simulink model "AsteroidImpact"  (R2021b)
settings: Solver=ode4  StartTime=0.0  StopTime=45  FixedStep=0.2  RelTol=1e-3
settings Model: Creator=KNMALE002  LastModifiedBy=lbaat
settings SolverCC: AlgebraicLoopSolver=TrustRegion
settings DataIOCC: SaveOutput=off  SignalLogging=off  DSMLogging=off  ReturnWorkspaceOutputs=off  TimeSaveName=simulation_time
settings DebuggingCC: SFMachineParentedDataDiag=warning  ArithmeticOperatorsInVariantConditions=warning
settings SFSimCC: CustomCodeUndefinedFunction=UseInterfaceOnly

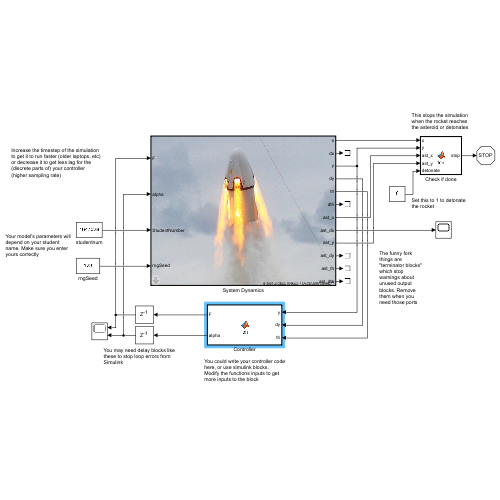
[thumbnail: Simulink's stored preview of the top-level diagram]
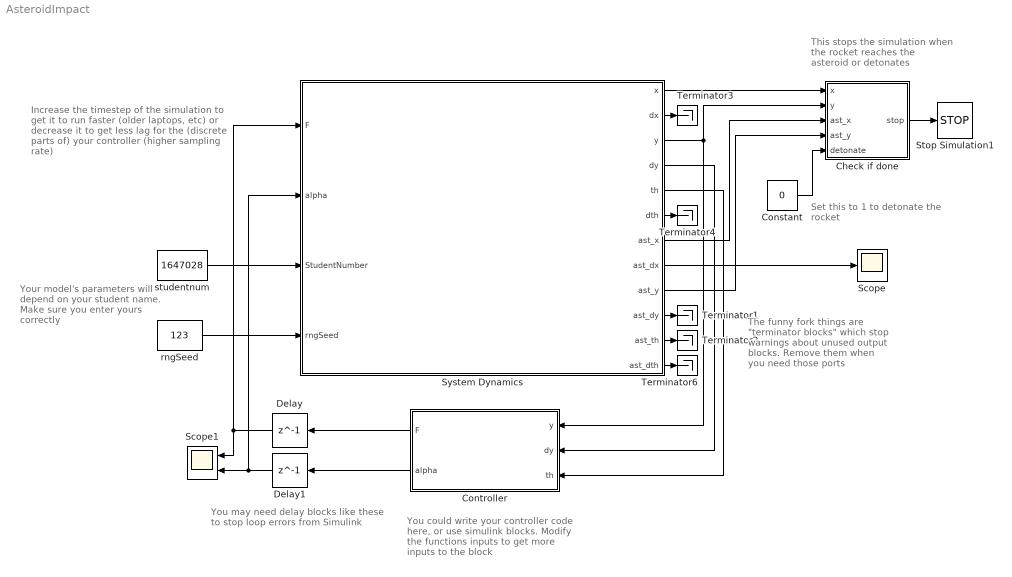
== system AsteroidImpact ==
  note: Increase the timestep of the simulation to get it to run faster (older laptops, etc) or decrease it to get less lag for the (discrete parts of) your controller (higher sampling rate)
  note: You may need delay blocks like these to stop loop errors from Simulink
  note: Your model's parameters will depend on your student name. Make sure you enter yours correctly
  note: You could write your controller code here, or use simulink blocks. Modify the functions inputs to get more inputs to the block
  note: The funny fork things are "terminator blocks" which stop warnings about unused output blocks. Remove them when you need those ports
  note: This stops the simulation when the rocket reaches the asteroid or detonates
  note: Set this to 1 to detonate the rocket
  Check if done : MATLAB Function  TreatAsAtomicUnit=on
  Constant : Constant  Value=0
  Controller : MATLAB Function  TreatAsAtomicUnit=on
  Delay : Delay  DelayLength=1  InitialCondition=10000000000
  Delay1 : Delay  DelayLength=1
  Scope : Scope
  Scope1 : Scope  NumInputPorts=2
  Stop Simulation1 : Stop
  System Dynamics : Subsystem  TreatAsAtomicUnit=on  mask{Value=1}
      mask prompts: Value "Enter mode (1, 2 or 3)"
      mask TypeOptions Value: ScenarioVar/Value
      mask Display: image('lander.jpg');
  Terminator{1..4,6} (5 alike) : Terminator
  rngSeed : Constant  Value=123
  studentnum : Constant  Value=1647028
  wires:
  studentnum/1 -> System Dynamics/3(StudentNumber)
  System Dynamics/1(x) -> Check if done/1(x)
  rngSeed/1 -> System Dynamics/4(rngSeed)
  System Dynamics/3(y) -> Check if done/2(y), Controller/1(y)
  System Dynamics/12(ast_dth) -> Terminator6/1
  System Dynamics/7(ast_x) -> Check if done/3(ast_x)
  System Dynamics/9(ast_y) -> Check if done/4(ast_y)
  System Dynamics/8(ast_dx) -> Scope/1
  System Dynamics/11(ast_th) -> Terminator2/1
  Check if done/1(stop) -> Stop Simulation1/1
  Delay1/1 -> Scope1/2, System Dynamics/2(alpha)
  Delay/1 -> Scope1/1, System Dynamics/1(F)
  Controller/1(F) -> Delay/1
  Controller/2(alpha) -> Delay1/1
  Constant/1 -> Check if done/5(detonate)
  System Dynamics/4(dy) -> Controller/2(dy)
  System Dynamics/5(th) -> Controller/3(th)
  System Dynamics/10(ast_dy) -> Terminator1/1
  System Dynamics/2(dx) -> Terminator3/1
  System Dynamics/6(dth) -> Terminator4/1

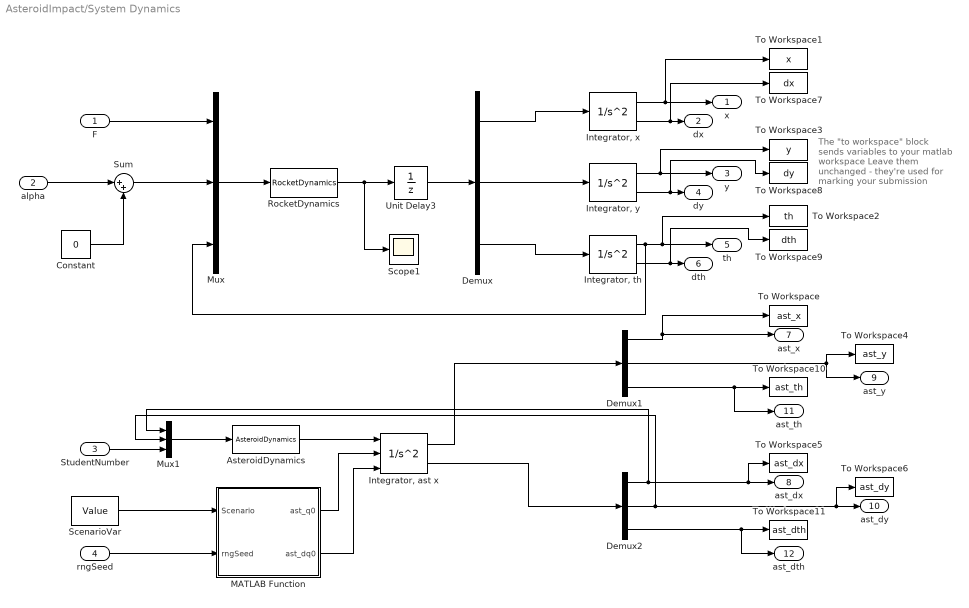
== system AsteroidImpact/System Dynamics ==
  note: The "to workspace" block sends variables to your matlab workspace
      |
      | Leave them unchanged - they're used for marking your submission
  F : Inport
  alpha : Inport  Port=2
  StudentNumber : Inport  Port=3
  rngSeed : Inport  Port=4
  AsteroidDynamics : MATLABFcn  MATLABFcn=AsteroidDynamics  OutputDimensions=3
  Constant : Constant  Value=0
  Demux : Demux  Outputs=3
  Demux1 : Demux  Outputs=3
  Demux2 : Demux  Outputs=3
  "Integrator, th" : SecondOrderIntegrator  ICX=0  ICDXDT=0
  "Integrator, x" : SecondOrderIntegrator  ICX=0
  "Integrator, y" : SecondOrderIntegrator  ICX=0
  "Integrator, ast x" : SecondOrderIntegrator  ICSourceX=external  ICX=x0  ICSourceDXDT=external
  MATLAB Function : MATLAB Function  TreatAsAtomicUnit=on
  Mux : Mux  Inputs=3
  Mux1 : Mux  Inputs=3
  RocketDynamics : MATLABFcn  MATLABFcn=RocketDynamics  Output1D=off
  ScenarioVar : Constant  Value=Value
  Scope1 : Scope
  Sum : Sum  Inputs=|++
  To Workspace : ToWorkspace  VariableName=ast_x  SampleTime=-1
  To Workspace1 : ToWorkspace  VariableName=x  SampleTime=-1
  To Workspace10 : ToWorkspace  VariableName=ast_th  SampleTime=-1
  To Workspace11 : ToWorkspace  VariableName=ast_dth  SampleTime=-1
  To Workspace2 : ToWorkspace  VariableName=th  SampleTime=-1
  To Workspace3 : ToWorkspace  VariableName=y  SampleTime=-1
  To Workspace4 : ToWorkspace  VariableName=ast_y  SampleTime=-1
  To Workspace5 : ToWorkspace  VariableName=ast_dx  SampleTime=-1
  To Workspace6 : ToWorkspace  VariableName=ast_dy  SampleTime=-1
  To Workspace7 : ToWorkspace  VariableName=dx  SampleTime=-1
  To Workspace8 : ToWorkspace  VariableName=dy  SampleTime=-1
  To Workspace9 : ToWorkspace  VariableName=dth  SampleTime=-1
  Unit Delay3 : UnitDelay  SampleTime=-1  HasFrameUpgradeWarning=on
  x : Outport  PortDimensions=1  VectorParamsAs1DForOutWhenUnconnected=off
  dx : Outport  Port=2  PortDimensions=1  VectorParamsAs1DForOutWhenUnconnected=off
  y : Outport  Port=3  PortDimensions=1  VectorParamsAs1DForOutWhenUnconnected=off
  dy : Outport  Port=4  PortDimensions=1  VectorParamsAs1DForOutWhenUnconnected=off
  th : Outport  Port=5  PortDimensions=1  VectorParamsAs1DForOutWhenUnconnected=off
  dth : Outport  Port=6  PortDimensions=1  VectorParamsAs1DForOutWhenUnconnected=off
  ast_x : Outport  Port=7  PortDimensions=1  VectorParamsAs1DForOutWhenUnconnected=off
  ast_dx : Outport  Port=8  PortDimensions=1  VectorParamsAs1DForOutWhenUnconnected=off
  ast_y : Outport  Port=9  PortDimensions=1  VectorParamsAs1DForOutWhenUnconnected=off
  ast_dy : Outport  Port=10  PortDimensions=1  VectorParamsAs1DForOutWhenUnconnected=off
  ast_th : Outport  Port=11  PortDimensions=1  VectorParamsAs1DForOutWhenUnconnected=off
  ast_dth : Outport  Port=12  PortDimensions=1  VectorParamsAs1DForOutWhenUnconnected=off
  wires:
  "Integrator, th"/1 -> th/1, To Workspace2/1, Mux/3
  Demux/1 -> "Integrator, x"/1
  Demux/2 -> "Integrator, y"/1
  Demux/3 -> "Integrator, th"/1
  "Integrator, x"/1 -> x/1, To Workspace1/1
  "Integrator, x"/2 -> To Workspace7/1, dx/1
  "Integrator, y"/2 -> To Workspace8/1, dy/1
  "Integrator, th"/2 -> To Workspace9/1, dth/1
  Mux/1 -> RocketDynamics/1
  rngSeed/1 -> MATLAB Function/2(rngSeed)
  ScenarioVar/1 -> MATLAB Function/1(Scenario)
  F/1 -> Mux/1
  alpha/1 -> Sum/1
  Demux1/2 -> To Workspace4/1, ast_y/1
  Demux1/3 -> To Workspace10/1, ast_th/1
  Demux2/3 -> ast_dth/1, To Workspace11/1
  Mux1/1 -> AsteroidDynamics/1
  AsteroidDynamics/1 -> "Integrator, ast x"/1
  "Integrator, ast x"/1 -> Demux1/1
  "Integrator, ast x"/2 -> Demux2/1
  Demux1/1 -> To Workspace/1, ast_x/1
  Demux2/1 -> Mux1/1, To Workspace5/1, ast_dx/1
  Demux2/2 -> Mux1/2, To Workspace6/1, ast_dy/1
  MATLAB Function/1(ast_q0) -> "Integrator, ast x"/2
  MATLAB Function/2(ast_dq0) -> "Integrator, ast x"/3
  StudentNumber/1 -> Mux1/3
  Unit Delay3/1 -> Demux/1
  "Integrator, y"/1 -> y/1, To Workspace3/1
  RocketDynamics/1 -> Scope1/1, Unit Delay3/1
  Constant/1 -> Sum/2
  Sum/1 -> Mux/2

== matlab function AsteroidImpact/System Dynamics/MATLAB Function ==
  data: ast_q0 output; ast_dq0 output; Scenario input; rngSeed input
function [ast_q0, ast_dq0] = fcn(Scenario, rngSeed)
rng(rngSeed);

if (Scenario == 1)
    x0 = -3000;
    y0 =  5000;
    th0 =   0;
    dx0 = 182;
    dy0 = 0;
    dth0 = 0;

elseif (Scenario == 2)
    x0 = -2000 + rand_within_plus_minus(100);
    y0 = 4000 + rand_within_plus_minus(100); 
    th0 = 0;
    dx0 = 170;
    dy0 = 0;
    dth0 = 0.1;

elseif (Scenario == 3)
    x0 = -2500;
    y0 = 3000;
    th0 = 0;
    dx0 = 160;
    dy0 = 100;
    dth0 = deg2rad(rand_within_plus_minus(20)); % rad/sec

else
    error('You entered an invalid mode -- make sure Scenario = 1, 2 or 3')
end

ast_q0  = [ x0;  y0;  th0];
ast_dq0 = [dx0; dy0; dth0];

end

% calling rand_within_plus_minus(100) returns a number between -100 and 100
function n = rand_within_plus_minus(interval)
    n = (rand - 0.5) * 2 * interval;
end

== matlab function AsteroidImpact/Controller ==
  data: F output; alpha output; y input; dy input; th input
function [F, alpha] = fcn(y, dy, th)

F = 1000000;
alpha = 0;

== matlab function AsteroidImpact/Check if done ==
  data: x input; stop output; y input; ast_x input; ast_y input; detonate input
function stop = fcn(x, y, ast_x, ast_y, detonate)
    % given the signal to detonate
    if detonate == 1
        stop = 1;

    % rocket has hit the asteroid
    elseif norm([x; y] - [ast_x; ast_y]) < 100
        stop = 1;
    
    % rocket has hit the ground OR asteroid is close to they city
    elseif y < 0 || ast_y < 200
        stop = 1;
    
    else
        stop = 0;
    end
end
